simulink model "mars_rover_ex_1b"  (R2023a)
settings: Solver=ode23t  StartTime=0.0  StopTime=Rover.simStopTimeEx1b  FixedStep=1e-2  MaxStep=0.1  RelTol=1e-3  AbsTol=1e-3  EnableMultiTasking=on
StartFcn:
  | mars_rover_ex1b_sim_callback
model workspace (MATLAB code in the model file):
  | addpath("mars_rover_helpers");
  | % Load Rover Arm model for IK
  | mdlpath = ['mars_rover_data',filesep,'mars_rover_arm'];
  | load_system(mdlpath);
  | 
  | imdata = zeros(3,3,3);
  | 
  | % Temp
  | Kp_steer = 1;
  | Ki_steer = 1;
  | Kd_steer = 1;
  | 
  | Kp = 1;
  | Ki = 1;
  | Kd = 1;
values from neighbouring files (symbols this model uses):
  cam_base_angle = 0    [mars_rover_params.m]
  cam_target_angle = 20    [mars_rover_params.m]
  mapData = false(197,200)    [mars_rover_params.m]    (also in mars_rover_startup.m)
  roverPath = app.rover_path    [NavigateOnMars.m]    (also in mars_rover_params.m = rover_path1)
undefined symbols (not defined in the file or in its folder): Arm, armJointAng, armJointTrqs, cameraData, eeConfig, pose, Rover, rover_path_ex1, sampleLocation, steerAng, steerTrqs, Terrain, vSpeed, Wheel1_G, Wheel2_G, Wheel3_G, Wheel4_G, Wheel5_G, Wheel6_G, wheelTrqs, wSpeeds, X, Y, Z
libraries: sm_lib x238, nesl_utility x80, slpidlib x3, simulink x3, simulink_extras x2, robotcorelib x1, robotalgslib x1
(part 1 of 9)
settings Model: PacingRate=4  Creator=The MathWorks, Inc.
settings SolverCC: AutoScaleAbsTol=off  ZeroCrossAlgorithm=Adaptive  AlgebraicLoopSolver=TrustRegion  MinimalZcImpactIntegration=on  MaxZcPerStep=1
settings DataIOCC: MaxDataPoints=10000  SaveFormat=Array  ReturnWorkspaceOutputsName=sm_mars_rover_out_ex1b
settings OptimizationCC: LifeSpan=inf
settings DebuggingCC: IgnoredZcDiagnostic=none  UnconnectedInputMsg=warning  UnconnectedOutputMsg=warning  UnconnectedLineMsg=warning  AllowSymbolicDim=off  SFUnexpectedBacktrackingDiag=warning  SFNoUnconditionalDefaultTransitionDiag=warning  SFExecutionAtInitializationDiag=none  ArithmeticOperatorsInVariantConditions=warning
settings ModelReferenceCC: EnableRefExpFcnMdlSchedulingChecks=on
settings SFSimCC: SimUseLocalCustomCode=off  CustomCodeUndefinedFunction=UseInterfaceOnly
settings RTWCC: RTWUseLocalCustomCode=off  DLArmComputeVersion=19.05
settings CodeAppCC: StateflowObjectComments=on
settings GRTTargetCC: TargetLangStandard=C89/C90 (ANSI)
settings ConfigComp: CovMetricSettings=dw  CovSaveCumulativeToWorkspaceVar=on  CovSaveSingleToWorkspaceVar=on  CovExternalEMLEnable=off  CovSFcnEnable=off
settings SimscapeCC: SimscapeLogType=all  SimscapeLogSimulationStatistics=on  SimscapeLogName=simlog_sm_mars_rover  SimscapeLogLimitData=off  SimscapeLogDataHistory=10000
settings DiagnosticsConfigSet: SimMechanicsUnconnectedFramePorts=none  SimMechanicsUnconnectedGeometryPorts=none  SimMechanicsConflictingReferenceFrames=none
settings ExplorerConfigSet: SimMechanicsOpenEditorOnUpdate=off  InternalSimMechanicsExplorerSettings="<ExplorerConfiguration><canonicalview>default</canonicalview><AnimationSetting><BasePlaybackSpeed>1.0</BasePlaybackSpeed><PlaybackSpeedFactor>16.0</PlaybackSpeedFactor></AnimationSetting><TilePanel><TileInfo><Tiles Columns=\"1\" Count=\"1\" Rows=\"1\"><Column Weight=\"1\"/><Row Weight=\"1\"/><Tile Height=\"1\" Width=\"1\" X=\"0\" Y=\"0\"/></Tiles></TileInfo><SceneInfo><SceneViewer><BGColor><R>0.819607853889465332</R><G>0.709803938865661621</G><B>0.662745118141174316</B></BGColor><Camera><DoPerspective>on</DoPerspective><Position><X>20.0000024966346217</X><Y>19.6116525700285997</Y><Z>47.9479667849964954</Z></Position><Center><X>20.0000024966346217</X><Y>19.6116525700285997</Y><Z>2.96310309448505915</Z></Center><Up><X>0</X><Y>1</Y><Z>-0</Z></Up><ViewLimDist>1</ViewLimDist><YLim>0.466307658154998583</YLim><XLim>0.817592760631764226</XLim></Camera></SceneViewer></SceneInfo></TilePanel><MechEditorPanel><Cameras><Camera><Id>Camera1</Id><Value><Name>Rover_Free_View</Name><NativeCamera><PositionKeyframeSet/><CenterKeyframeSet/><UpVectorKeyframeSet/></NativeCamera></Value></Camera><Camera><Id>Camera6</Id><Value><Name>Rover_Right_ViewA</Name><NativeCamera><PositionTrackingFeature>Mars_Rover.Rover_Plant_Model_And_Control.Rover.Chassis.Chasis_Camera_RightA.R</PositionTrackingFeature><CenterTrackingFeature>Mars_Rover.Rover_Plant_Model_And_Control.Rover.Chassis.Chasis_Camera_RightA.R</CenterTrackingFeature><UpVectorTrackingFeature>Mars_Rover.Rover_Plant_Model_And_Control.Rover.Chassis.Chasis_Camera_RightA.R</UpVectorTrackingFeature><CenterTrackingOrigin>off</CenterTrackingOrigin><CenterTrackingDirection>+X</CenterTrackingDirection><UpVectorTrackingDirection>+Z</UpVectorTrackingDirection></NativeCamera></Value></Camera><Camera><Id>Camera7</Id><Value><Name>Rover_Rear_View</Name><NativeCamera><PositionTrackingFeature>Mars_Rover.Rover_Plant_Model_And_Control.Rover.Chassis.Chasis_Camera_Rear.R</PositionTrackingFeature><CenterTrackingFeature>Mars_Rover.Rover_Plant_Model_And_Control.Rover.Chassis.Chasis_Camera_Rear.R</CenterTrackingFeature><UpVectorTrackingFeature>Mars_Rover.Rover_Plant_Model_And_Control.Rover.Chassis.Chasis_Camera_Rear.R</UpVectorTrackingFeature><CenterTrackingOrigin>off</CenterTrackingOrigin><CenterTrackingDirection>-Y</CenterTrackingDirection><UpVectorTrackingDirection>+Z</UpVectorTrackingDirection></NativeCamera></Value></Camera><Camera><Id>Camera8</Id><Value><Name>Rover_Top_View</Name><NativeCamera><PositionTrackingFeature>Mars_Rover.Rover_Plant_Model_And_Control.Rover.Chassis.Chasis_Camera_Top.R</PositionTrackingFeature><CenterTrackingFeature>Mars_Rover.Rover_Plant_Model_And_Control.Rover.Chassis.Chasis_Camera_Top.R</CenterTrackingFeature><UpVectorTrackingFeature>Mars_Rover.Rover_Plant_Model_And_Control.Rover.Chassis.Chasis_Camera_Top.R</UpVectorTrackingFeature><CenterTrackingOrigin>off</CenterTrackingOrigin><CenterTrackingDirection>-Z</CenterTrackingDirection><UpVectorTrackingDirection>+X</UpVectorTrackingDirection></NativeCamera></Value></Camera><Camera><Id>Camera9</Id><Value><Name>Rover_Right_ViewB</Name><NativeCamera><PositionTrackingFeature>Mars_Rover.Rover_Plant_Model_And_Control.Rover.Chassis.Chasis_Camera_RightB.R</PositionTrackingFeature><CenterTrackingFeature>Mars_Rover.Rover_Plant_Model_And_Control.Rover.Chassis.Chasis_Camera_RightB.R</CenterTrackingFeature><UpVectorTrackingFeature>Mars_Rover.Rover_Plant_Model_And_Control.Rover.Chassis.Chasis_Camera_RightB.R</UpVectorTrackingFeature><CenterTrackingOrigin>off</CenterTrackingOrigin><CenterTrackingDirection>+X</CenterTrackingDirection><UpVectorTrackingDirection>+Z</UpVectorTrackingDirection></NativeCamera></Value></Camera><Camera><Id>Camera10</Id><Value><Name>RoverNavCamL</Name><NativeCamera><PositionTrackingFeature>Mars_Rover.Rover_Plant_Model_And_Control.Rover.Camera.rsm_head_1_RIGID.CameraFrameL.F</PositionTrackingFeature><CenterTrackingFeature>Mars_Rover.Rover_Plant_Model_And_Control.Rover.Camera.rsm_head_1_RIGID.CameraFrameL.F</CenterTrackingFeature><UpVectorTrackingFeature>Mars_Rover.Rover_Plant_Model_And_Control.Rover.Camera.rsm_head_1_RIGID.CameraFrameL.F</UpVectorTrackingFeature><CenterTrackingOrigin>off</CenterTrackingOrigin><CenterTrackingDirection>+X</CenterTrackingDirection><UpVectorTrackingDirection>+Z</UpVectorTrackingDirection></NativeCamera></Value></Camera><Camera><Id>Camera11</Id><Value><Name>RoverNavCamR</Name><NativeCamera><PositionTrackingFeature>Mars_Rover.Rover_Plant_Model_And_Control.Rover.Camera.rsm_head_1_RIGID.CameraFrameR.F</PositionTrackingFeature><CenterTrackingFeature>Mars_Rover.Rover_Plant_Model_And_Control.Rover.Camera.rsm_head_1_RIGID.CameraFrameR.F</CenterTrackingFeature><UpVectorTrackingFeature>Mars_Rover.Rover_Plant_Model_And_Control.Rover.Camera.rsm_head_1_RIGID.CameraFrameR.F</UpVectorTrackingFeature><CenterTrackingOrigin>off</CenterTrackingOrigin><CenterTrackingDirection>+X</CenterTrackingDirection><UpVectorTrackingDirection>+Z</UpVectorTrackingDirection></NativeCamera></Value></Camera></Cameras><GfxPanelCameraMap><MapElement CameraMLId=\"Camera10\" GfxPanelIndex=\"0\"/></GfxPanelCameraMap><VideoCreator><PlaybackSpeedRatio>8</PlaybackSpeedRatio><FrameRate>30</FrameRate><VideoFormat>MPEG-4</VideoFormat><FrameSize>[800 600]</FrameSize></VideoCreator></MechEditorPanel></ExplorerConfiguration>"

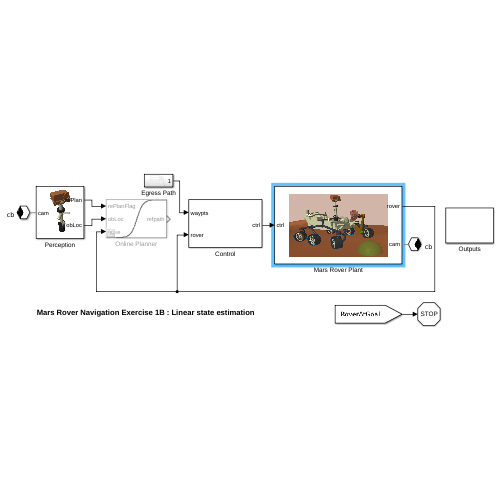
[thumbnail: Simulink's stored preview of the top-level diagram]
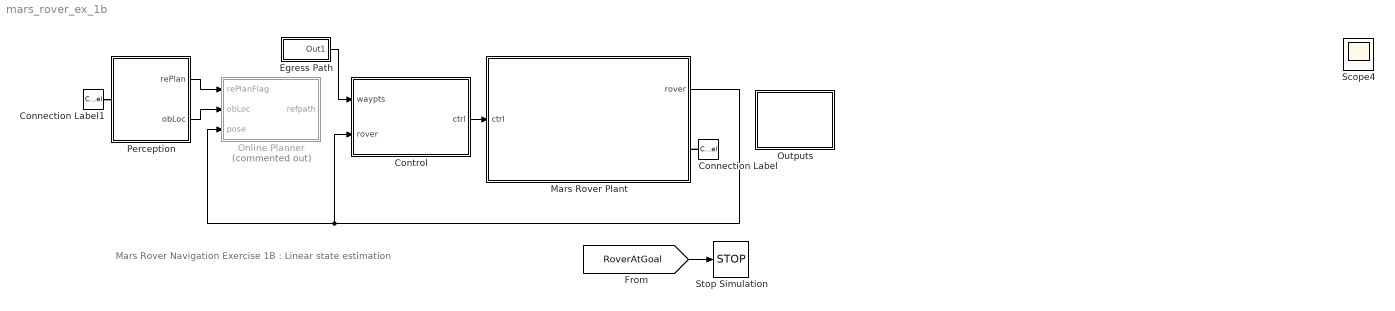
== system mars_rover_ex_1b ==
  note: Mars Rover Navigation Exercise 1B : Linear state estimation
  Connection Label : ConnectionLabel  Label=cb
  Connection Label1 : ConnectionLabel  Label=cb
  Control : Subsystem
  Egress Path : Subsystem
  Mars Rover Plant : Subsystem
      mask Display: image('$imagefile'); % Use "Edit Image" on toolstrip to change.
  Online Planner : Subsystem  Commented=on
      mask Display:
      | x = -5:0.01:5;
      | y = tanh(x);
      | plot(x,y)
  Outputs : Subsystem
  Perception : Subsystem
      mask Display: image('$imagefile'); % Use "Edit Image" on toolstrip to change.
  Stop Simulation : Stop
  Scope4 : Scope
  wires:
  Mars Rover Plant/1(rover) -> Online Planner/3(pose), Control/2(rover)
  Control/1(ctrl) -> Mars Rover Plant/1(ctrl)
  Perception/1(rePlan) -> Online Planner/1(rePlanFlag)
  Perception/2(obLoc) -> Online Planner/2(obLoc)
  Egress Path/1(Out1) -> Control/1(waypts)
  [RoverAtGoal] -> Stop Simulation/1
  connections:
  Connection Label/LConn1 -- Mars Rover Plant/RConn1
  Connection Label1/LConn1 -- Perception/LConn1

== system mars_rover_ex_1b/Control ==
  waypts : Inport
  rover : Inport  Port=2
  Bus Creator : BusCreator  Inputs=steerTrqs,wheelTrqs,armJointTrqs
  Bus Selector : BusSelector  OutputSignals=pose,vSpeed,steerAng,wSpeeds,sampleLocation,armJointAng
  Manipulator Control : Subsystem  Commented=on
  Rover Control : Subsystem
  ctrl : Outport
  wires:
  Bus Selector/3 -> Rover Control/4(ActSteerAng)  "<steerAng>"
  Bus Selector/6 -> Manipulator Control/2(ActJointAngles)  "<armJointAng>"
  Bus Selector/5 -> Manipulator Control/1(SampleLocation)  "<sampleLocation>"
  Bus Selector/2 -> Rover Control/3(vSpeed)  "<vSpeed>"
  Rover Control/2(WheelTrqs) -> Bus Creator/2  "wheelTrqs"
  Bus Selector/1 -> Rover Control/2(CurrentPose)  "<pose>"
  Bus Selector/4 -> Rover Control/5(ActWheelSpeed)  "<wSpeeds>"
  Rover Control/1(SteerTrqs) -> Bus Creator/1  "steerTrqs"
  Manipulator Control/1(y) -> Bus Creator/3  "armJointTrqs"
  rover/1 -> Bus Selector/1
  waypts/1 -> Rover Control/1(WayPts)
  Bus Creator/1 -> ctrl/1

== system mars_rover_ex_1b/Egress Path ==
  Constant : Constant  Value=rover_path_ex1.x
  Constant1 : Constant  Value=rover_path_ex1.y
  Matrix Concatenate : Concatenate  Mode=Multidimensional array  ConcatenateDimension=2
  Out1 : Outport
  wires:
  Constant/1 -> Matrix Concatenate/1
  Constant1/1 -> Matrix Concatenate/2
  Matrix Concatenate/1 -> Out1/1

== system mars_rover_ex_1b/Mars Rover Plant ==
  ctrl : Inport
  Bus Creator : BusCreator  Inputs=pose,vSpeed,steerAng,wSpeeds,armJointAng,sampleLocation
  Bus Selector : BusSelector  OutputSignals=steerTrqs,wheelTrqs,armJointTrqs
  DesRoverPathViz : Subsystem
  Manipulator Plant Model : Subsystem  Commented=on
      settings: PortSchema="{\"entries\":[{\"content\":{\"sides\":[{\"content\":{\"connectorIds\":[\"LConn1\",\"In1\"]},\"type\":\"ConnectorPlacement.EquallySpacedRectSide\",\"uuid\":\"1d5d5bba-8fe4-4512-81c9-941bf10e7a7e\"},{\"content\":{\"connectorIds\":[\"RConn1\",\"RConn2\",\"Out1\",\"Out2\"],\"side\":\"RIGHT\"},\"type\":\"ConnectorPlacement.EquallySpacedRectSide\",\"uuid\":\"9a182200-9de3-47d0-8b03-f46c5c0d90b9\"},{\"content\":{\"connectorIds\":[],\"side\":\"TOP\"},\"type\":\"ConnectorPlacement.EquallySpacedRectSide\",\"uuid\":\"d91c9a9a-8a5e-48c7-bbfb-96bbdec144af\"}]},\"type\":\"ConnectorPlacement.EquallySpacedConnector\",\"uuid\":\"893c2cf1-507c-408d-8167-3b555343645b\"}],\"packageUris\":[\"http://schema.mathworks.com/mf0/Connector/R2020b\"],\"version\":\"1.0\"}"
      mask Display:
      | image('RoverArmIcon.png'); % Use "Edit Image" on toolstrip to change.
      | 
      | color('black');
      | port_label('RConn',1,' sd','interpreter','tex')
      | port_label('LConn',1,' sb','interpreter','tex')
      | port_label('RConn',2,' armB','interpreter','tex')
      | port_label('output', 1, 'angles');
      | port_label('output', 2, 'sample');
      | port_label('input', 1, 'trqs');
  Rover Plant Model : Subsystem
      mask Display:
      | image('RoverIcon.PNG');
      | %image('$imagefile'); % Use "Edit Image" on toolstrip to change.
      | 
      | color('black');
      | port_label('LConn',1,' ref','interpreter','tex')
      | port_label('RConn',1,' armB','interpreter','tex')
      | port_label('RConn',2,' SD','interpreter','tex')
      | port_label('RConn',3,' CB','interpreter','tex')
      | port_label('output', 1, 'pose');
      | port_label('output', 2, 'vSpeed');
      | port_label('output', 3, 'sAng');
      | port_label('output', 4, 'wSpeed');
      | port_label('input', 1, 'sTrqs');
      | port_label('input', 2, 'wTrqs');
  cam : PMIOPort  Side=Right
  rover : Outport
  wires:
  Bus Selector/1 -> Rover Plant Model/1(Input)  "<steerTrqs>"
  Bus Selector/2 -> Rover Plant Model/2(Input1)  "<wheelTrqs>"
  Rover Plant Model/1(Pose) -> Bus Creator/1  "pose"
  Rover Plant Model/2(actRoverSpeed) -> Bus Creator/2  "vSpeed"
  Rover Plant Model/4(actWheelSpeeds) -> Bus Creator/4  "wSpeeds"
  Manipulator Plant Model/1(armJointAng) -> Bus Creator/5  "armJointAng"
  Manipulator Plant Model/2(sampleLocation) -> Bus Creator/6  "sampleLocation"
  Bus Selector/3 -> Manipulator Plant Model/1(Input)  "<armJointTrqs>"
  Bus Creator/1 -> rover/1
  Rover Plant Model/3(actSteerAng) -> Bus Creator/3  "steerAng"
  ctrl/1 -> Bus Selector/1
  connections:
  Rover Plant Model/LConn1 -- Manipulator Plant Model/LConn1 -- DesRoverPathViz/LConn1
  Rover Plant Model/RConn1 -- Manipulator Plant Model/RConn2
  Rover Plant Model/RConn2 -- Manipulator Plant Model/RConn1
  cam/RConn1 -- Rover Plant Model/RConn3

== system mars_rover_ex_1b/Online Planner ==
  rePlanFlag : Inport
  obLoc : Inport  Port=2
  pose : Inport  Port=3
  Bus Selector : BusSelector  OutputSignals=pose
  Constant13 : Constant  Value=[roverPath.x(end) roverPath.y(end) 0]
  Constant2 : Constant  Value=[roverPath.x roverPath.y]
  Online Planner : Subsystem
  Triggered Subsystem1 : Subsystem  TreatAsAtomicUnit=on
  Unit Delay : UnitDelay  InitialCondition=mapData  SampleTime=-1  HasFrameUpgradeWarning=on
  refpath : Outport
  tag scope: RefPath=global, mapData=global
  wires:
  Constant13/1 -> Online Planner/3(endLocation)
  Unit Delay/1 -> Online Planner/1(mapData)
  rePlanFlag/1 -> Triggered Subsystem1/Trigger, Online Planner/Trigger
  Triggered Subsystem1/1(Out1) -> Online Planner/2(startLocation)
  Online Planner/1(refpath) -> [RefPath], refpath/1
  pose/1 -> Bus Selector/1
  Bus Selector/1 -> Triggered Subsystem1/1(startLocation)  "<pose>"
  Constant2/1 -> Online Planner/5(initialRoverPath)
  Online Planner/2(newMapData) -> Unit Delay/1, [mapData]
  obLoc/1 -> Online Planner/4(obstacleLocation)

== system mars_rover_ex_1b/Outputs ==
  Rover Outputs : Subsystem

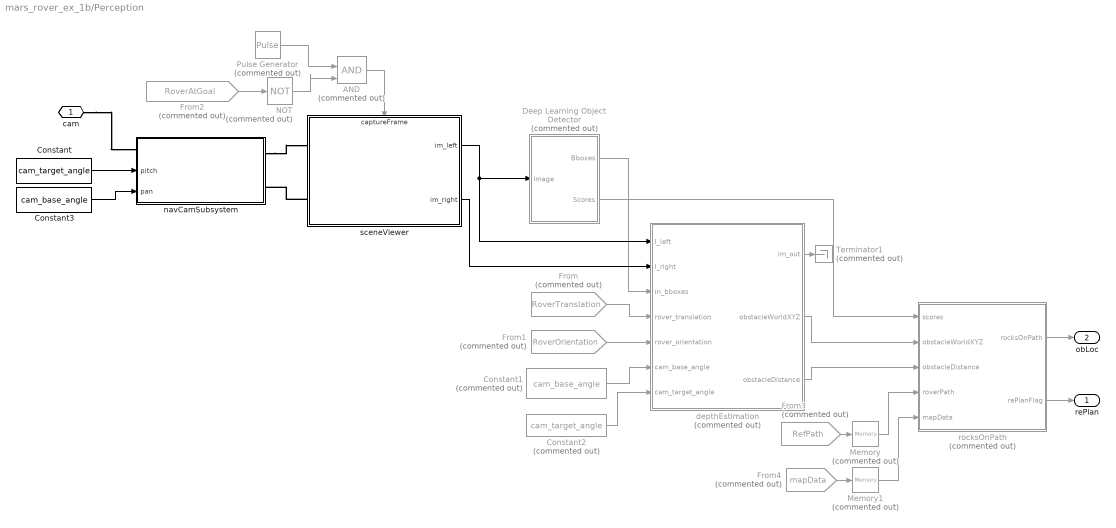
== system mars_rover_ex_1b/Perception ==
  AND : Logic  Commented=on  IconShape=distinctive  AllPortsSameDT=off  OutDataTypeStr=boolean
  Constant : Constant  Value=cam_target_angle
  Constant1 : Constant  Commented=on  Value=cam_base_angle
  Constant2 : Constant  Commented=on  Value=cam_target_angle
  Constant3 : Constant  Value=cam_base_angle
  Deep Learning Object Detector : Subsystem  Commented=on  mask(Deep Learning Object Detector){Detector=Detector from MAT-file, DetectorFunction=untitled, DetectorFilePath=rockDetectorDL.mat, MaxDetections=500, Bboxes=on, Labels=off, Scores=on, UseROI=off, ROI=[1 1 100 100], Threshold=0.8, NumStrongestRegions=2000, UseMinSize=off, MinSize=[1 1], UseMaxSize=off, MaxSize=[50 50], ForceInterpretedSim=off}
      mask prompts: Detector "vision:ObjectDetectorBlock:Detector"; DetectorFunction "vision:ObjectDetectorBlock:MatlabFunction"; DetectorFilePath "vision:ObjectDetectorBlock:FilePath"; MaxDetections "vision:ObjectDetectorBlock:MaxDetections"; Bboxes "vision:ObjectDetectorBlock:Bboxes"; Labels "vision:ObjectDetectorBlock:Labels"; Scores "vision:ObjectDetectorBlock:Scores"; UseROI "vision:ObjectDetectorBlock:UseROI"; Threshold "vision:ObjectDetectorBlock:Threshold"; NumStrongestRegions "vision:ObjectDetectorBlock:NumStrongestRegions"; UseMinSize "vision:ObjectDetectorBlock:UseMinSize"; UseMaxSize "vision:ObjectDetectorBlock:UseMaxSize"; ForceInterpretedSim "vision:ObjectDetectorBlock:ForceInterpretedSim"
      mask help: vision:ObjectDetectorBlock:Description
      mask init:
      | vision.internal.blocks.objectDetectorBlockWrapper(...
      |     'deep.blocks.internal.configureObjectDetector', ...
      |     gcb, ...
      |     bdroot, ...
      |     Detector, ...
      |     DetectorFilePath, ...
      |     DetectorFunction, ...
      |     logical(UseROI), ...
      |     ROI, ...
      |     Threshold, ...
      |     NumStrongestRegions, ...
      |     logical(UseMinSize), ...
      |     MinSize, ...
      |     logical(UseMaxSize), ...
      |     MaxSize, ...
      |     MaxDetections, ...
      |     logical(Bboxes), ...
      |     logical(Labels), ...
      |     logical(Scores), ...
      |     logical(ForceInterpretedSim));
      mask Help: helpview('vision', 'nnet_model_detect')
      mask TypeOptions Detector: vision:ObjectDetectorBlock:DetectorFromMatFile | vision:ObjectDetectorBlock:DetectorFromFunction
      mask Callback Detector: vision.internal.blocks.objectDetectorBlockWrapper('deep.blocks.internal.setNetworkSelectVisibility',gcb);
      mask Callback DetectorFunction: vision.internal.blocks.objectDetectorBlockWrapper('deep.blocks.internal.setObjectDetectorOptionsVisibility', gcb);
      mask Callback DetectorFilePath: vision.internal.blocks.objectDetectorBlockWrapper('deep.blocks.internal.setObjectDetectorOptionsVisibility', gcb);
      mask Callback UseROI: vision.internal.blocks.objectDetectorBlockWrapper('deep.blocks.internal.setEnabledParameterVisibility', gcb, 'UseROI', 'ROI');
      mask Callback UseMinSize: vision.internal.blocks.objectDetectorBlockWrapper('deep.blocks.internal.setEnabledParameterVisibility', gcb, 'UseMinSize', 'MinSize');
      mask Callback UseMaxSize: vision.internal.blocks.objectDetectorBlockWrapper('deep.blocks.internal.setEnabledParameterVisibility', gcb, 'UseMaxSize', 'MaxSize');
      mask DialogControl Detector Prompt: Detector:
      mask DialogControl DetectorFunction Prompt: MATLAB function:
      mask DialogControl DetectorFilePath Prompt: File path:
      mask DialogControl BrowseButton Prompt: vision:ObjectDetectorBlock:Browse
      mask DialogControl BrowseButton Callback: vision.internal.blocks.objectDetectorBlockWrapper('deep.blocks.internal.handleBrowseButtonClick', gcb);
      mask DialogControl OutputsTab Prompt: vision:ObjectDetectorBlock:Outputs
      mask DialogControl OutputsSizeGroup Prompt: vision:ObjectDetectorBlock:OutputsSize
      mask DialogControl MaxDetections Prompt: Maximum number of detections:
      mask DialogControl OutputPortsGroup Prompt: vision:ObjectDetectorBlock:OutputPorts
      mask DialogControl Bboxes Prompt: Bounding boxes
      mask DialogControl AdvancedTab Prompt: vision:ObjectDetectorBlock:Advanced
      mask DialogControl AdvancedParametersGroup Prompt: vision:ObjectDetectorBlock:AdvancedParameters
      mask DialogControl UseROI Prompt: Specify region of interest
      mask DialogControl Threshold Prompt: Detection threshold:
      mask DialogControl NumStrongestRegions Prompt: Number of strongest regions:
      mask DialogControl UseMinSize Prompt: Specify minimum region size
      mask DialogControl UseMaxSize Prompt: Specify maximum region size
      mask DialogControl HiddenContainer Prompt: Hidden Parameters
      mask DialogControl ForceInterpretedSim Prompt: Force interpreted simulation
  From : From  Commented=on  GotoTag=RoverTranslation  TagVisibility=global
  From1 : From  Commented=on  GotoTag=RoverOrientation  TagVisibility=global
  From2 : From  Commented=on  GotoTag=RoverAtGoal  TagVisibility=global
  From3 : From  Commented=on  GotoTag=RefPath  TagVisibility=global
  From4 : From  Commented=on  GotoTag=mapData  TagVisibility=global
  Memory : Memory  Commented=on  InitialCondition=[roverPath.x roverPath.y]
  Memory1 : Memory  Commented=on  InitialCondition=mapData
  NOT : Logic  Commented=on  Operator=NOT  IconShape=distinctive  AllPortsSameDT=off  OutDataTypeStr=boolean
  Pulse Generator : DiscretePulseGenerator  Commented=on  PulseType=Time based  Period=10000
  Terminator1 : Terminator  Commented=on
  depthEstimation : MATLAB Function  Commented=on  TreatAsAtomicUnit=on
  navCamSubsystem : Subsystem
      settings: PortSchema="{\"entries\":[{\"content\":{\"sides\":[{\"content\":{\"connectorIds\":[\"LConn1\",\"In1\",\"In2\"]},\"type\":\"ConnectorPlacement.EquallySpacedRectSide\",\"uuid\":\"2deb6c0b-0fb4-445b-86e3-b1fc7203c2ed\"},{\"content\":{\"connectorIds\":[\"RConn1\",\"RConn2\"],\"side\":\"RIGHT\"},\"type\":\"ConnectorPlacement.EquallySpacedRectSide\",\"uuid\":\"96d5d272-26bd-434a-b8d4-4dbdb87bfabc\"},{\"content\":{\"connectorIds\":[],\"side\":\"TOP\"},\"type\":\"ConnectorPlacement.EquallySpacedRectSide\",\"uuid\":\"0dc7d8f3-f281-4d7b-afc7-28fa8d470391\"}]},\"type\":\"ConnectorPlacement.EquallySpacedConnector\",\"uuid\":\"c3c449fe-5a97-4f9a-be85-0bfbae61164d\"}],\"packageUris\":[\"http://schema.mathworks.com/mf0/Connector/R2020b\"],\"version\":\"1.0\"}"
  rocksOnPath : MATLAB Function  Commented=on  TreatAsAtomicUnit=on
  sceneViewer : Subsystem
      settings: PortSchema="{\"entries\":[{\"content\":{\"sides\":[{\"content\":{\"connectorIds\":[\"LConn1\",\"LConn2\"]},\"type\":\"ConnectorPlacement.EquallySpacedRectSide\",\"uuid\":\"3e389f59-5740-42d0-b219-868887290247\"},{\"content\":{\"connectorIds\":[\"Out1\",\"Out2\"],\"side\":\"RIGHT\"},\"type\":\"ConnectorPlacement.EquallySpacedRectSide\",\"uuid\":\"8071baf0-f328-4328-afc3-7bbca75f94e9\"},{\"content\":{\"connectorIds\":[\"In1\"],\"side\":\"TOP\"},\"type\":\"ConnectorPlacement.EquallySpacedRectSide\",\"uuid\":\"389ad39b-6a15-4fbe-92ae-3d1bb225264a\"}]},\"type\":\"ConnectorPlacement.EquallySpacedConnector\",\"uuid\":\"9ad84bbc-3c32-4f8f-82ec-510eaa24821f\"}],\"packageUris\":[\"http://schema.mathworks.com/mf0/Connector/R2020b\"],\"version\":\"1.0\"}"
  cam : PMIOPort  Side=Left
  rePlan : Outport
  obLoc : Outport  Port=2
  wires:
  Deep Learning Object Detector/1(Bboxes) -> depthEstimation/3(in_bboxes)
  depthEstimation/2(obstacleWorldXYZ) -> rocksOnPath/2(obstacleWorldXYZ)
  depthEstimation/1(im_out) -> Terminator1/1
  From/1 -> depthEstimation/4(rover_translation)
  From1/1 -> depthEstimation/5(rover_orientation)
  Constant1/1 -> depthEstimation/6(cam_base_angle)
  Constant2/1 -> depthEstimation/7(cam_target_angle)
  From2/1 -> NOT/1
  NOT/1 -> AND/2
  rocksOnPath/1(rocksOnPath) -> obLoc/1
  rocksOnPath/2(rePlanFlag) -> rePlan/1
  Pulse Generator/1 -> AND/1
  From3/1 -> Memory/1
  Memory/1 -> rocksOnPath/4(roverPath)
  From4/1 -> Memory1/1
  Memory1/1 -> rocksOnPath/5(mapData)
  depthEstimation/3(obstacleDistance) -> rocksOnPath/3(obstacleDistance)
  Deep Learning Object Detector/2(Scores) -> rocksOnPath/1(scores)
  sceneViewer/1(im_left) -> Deep Learning Object Detector/1(Image), depthEstimation/1(I_left)
  AND/1 -> sceneViewer/1(captureFrame)
  sceneViewer/2(im_right) -> depthEstimation/2(I_right)
  Constant/1 -> navCamSubsystem/1(pitch)
  Constant3/1 -> navCamSubsystem/2(pan)
  connections:
  navCamSubsystem/RConn1 -- sceneViewer/LConn1
  sceneViewer/LConn2 -- navCamSubsystem/RConn2
  cam/RConn1 -- navCamSubsystem/LConn1

== system mars_rover_ex_1b/Control/Manipulator Control ==
  SampleLocation : Inport
  ActJointAngles : Inport  Port=2
  " Trajectory Planner" : Subsystem
  Add : Sum  Inputs=+-
  PID Control : slpidlib/PID Controller  Controller=PID  Form=Parallel  TimeDomain=Continuous-time  UseExternalTs=off  SampleTime=-1  IntegratorMethod=Forward Euler  FilterMethod=Forward Euler  ControllerParametersSource=internal  P=Arm.Kp_arm  I=Arm.Ki_arm  UseKiTs=off  D=Arm.Kd_arm  N=100  UseFilter=on  TunerSelectOption=Transfer Function Based (PID Tuner App)  InitialConditionSource=internal  InitialConditionForIntegrator=0  InitialConditionForFilter=0  DifferentiatorICPrevScaledInput=0  ExternalReset=none  TrackingMode=off  Kt=1  LimitOutput=off  SatLimitsSource=internal  UpperSaturationLimit=inf  LowerSaturationLimit=-inf  LinearizeAsGain=on  AntiWindupMode=none  Kb=1  POutMin=[]  POutMax=[]  IOutMin=[]  IOutMax=[]  DOutMin=[]  DOutMax=[]  NOutMin=[]  NOutMax=[]  SumOutMin=[]  SumOutMax=[]  SaturationOutMin=[]  SaturationOutMax=[]  PParamMin=[]  PParamMax=[]  IParamMin=[]  IParamMax=[]  DParamMin=[]  DParamMax=[]  NParamMin=[]  NParamMax=[]  KbParamMin=[]  KbParamMax=[]  KtParamMin=[]  KtParamMax=[]  KbOutMin=[]  KbOutMax=[]  KtOutMin=[]  KtOutMax=[]  IntegratorOutMin=[]  IntegratorOutMax=[]  FilterOutMin=[]  FilterOutMax=[]  SumI1OutMin=[]  SumI1OutMax=[]  SumI2OutMin=[]  SumI2OutMax=[]  SumI3OutMin=[]  SumI3OutMax=[]  SumI4OutMin=[]  SumI4OutMax=[]  SumDOutMin=[]  SumDOutMax=[]  DifferentiatorOutMin=[]  DifferentiatorOutMax=[]  FilterDiffOutCoefMin=[]  FilterDiffOutCoefMax=[]  ReciprocalOutMin=[]  ReciprocalOutMax=[]  SumDenOutMin=[]  SumDenOutMax=[]  SumNumOutMin=[]  SumNumOutMax=[]  DivideOutMin=[]  DivideOutMax=[]  UdiffTsProdOutMin=[]  UdiffTsProdOutMax=[]  NTsProdOutMin=[]  NTsProdOutMax=[]  UintegralTsProdOutMin=[]  UintegralTsProdOutMax=[]  UngainTsProdOutMin=[]  UngainTsProdOutMax=[]  IntegratorContinuousStateAttributes=''  IntegratorStateMustResolveToSignalObject=off  IntegratorRTWStateStorageClass=Auto  FilterContinuousStateAttributes=''  FilterStateMustResolveToSignalObject=off  FilterRTWStateStorageClass=Auto  ParallelPVariant=InternalParameters  IdealPVariant=Disabled  IVariant=InternalParameters  DVariant=InternalParameters  IntegratorVariant=Continuous  SatVariant=Disabled  AWVariant=Passthrough  PCopyVariant=Disabled  TRVariant=Disabled  FdbkBlocksVariant=Forward  IdealPFdbkVariant=Disabled  SatFdbkVariant=Disabled  DerivativeFilterVariant=ContFilter  NVariant=InternalParameters  NCopyVariant=Disabled  FilterICVariant=InternalICsFilter  IntegratorICVariant=InternalICs  ExternalResetVariant=Disabled  TRSumVariant=Passthrough  SumFdbkVariant=Disabled  SumVariant=Sum_PID  TsampFilterVariant=InternalTs  TsampNgainVariant=Passthrough  TsampIntegralVariant=Passthrough  ExternalSaturationOutDataTypeStr=Inherit: Same as second input
  y : Outport
  tag scope: ActJointAngles=global, DesiredJointAngles=global, JointActuatorTrqs=global
  wires:
  PID Control/1 -> y/1, [JointActuatorTrqs]
  SampleLocation/1 -> " Trajectory Planner"/1(SampleLocation)
  ActJointAngles/1 -> Add/2, [ActJointAngles], " Trajectory Planner"/2(ActJointAngles)
  " Trajectory Planner"/1(DesiredJointAngles) -> Add/1, [DesiredJointAngles]
  Add/1 -> PID Control/1

== system mars_rover_ex_1b/Control/Rover Control ==
  WayPts : Inport
  CurrentPose : Inport  Port=2
  vSpeed : Inport  Port=3
  ActSteerAng : Inport  Port=4
  ActWheelSpeed : Inport  Port=5
  Rover Path Planning And Control : Subsystem
  Steering Controller : Subsystem
  Wheel Speed Controller : Subsystem
  SteerTrqs : Outport
  WheelTrqs : Outport  Port=2
  wires:
  Rover Path Planning And Control/2(DesWheelSpeeds) -> Wheel Speed Controller/1(DesWheelSpeeds)
  ActWheelSpeed/1 -> Wheel Speed Controller/2(ActWheelSpeed)
  Rover Path Planning And Control/1(DesSteerAngs) -> Steering Controller/1(DesSteerAng)
  CurrentPose/1 -> Rover Path Planning And Control/2(CurrentPose)
  Steering Controller/1(SteerTrqs) -> SteerTrqs/1
  ActSteerAng/1 -> Steering Controller/2(ActSteerAng)
  vSpeed/1 -> Rover Path Planning And Control/3(vSpeed)
  Wheel Speed Controller/1(WheelTrqs) -> WheelTrqs/1
  WayPts/1 -> Rover Path Planning And Control/1(WayPts)

== system mars_rover_ex_1b/Mars Rover Plant/DesRoverPathViz ==
  Cylindrical Solid : sm_lib/Body Elements/Cylindrical Solid  Commented=on  GraphicAmbientColor=[0.15 0.15 0.15 1.0]  BasedOnType=Density  CenterOfMass=[0 0 0]  CenterOfMassUnits=m  GraphicDiffuseColor=[0.4 0.4 1.0]  CylinderLength=0.1  CylinderLengthUnits=m  CylinderRadius=1  CylinderRadiusUnits=m  Density=1000  DensityUnits=kg/m^3  DoExposeReferenceFrame=on  GraphicEmissiveColor=[0.0 0.0 0.0 1.0]  ExportEntireGeometry=off  SerializedFrames=<Frames/>  MarkerShape=Sphere  MarkerSize=10  GraphicType=FromGeometry  InertiaType=CalculateFromGeometry  Mass=1  MassUnits=kg  MomentsOfInertia=[1 1 1]  MomentsOfInertiaUnits=kg*m^2  GraphicOpacity=0.5  ProductsOfInertia=[0 0 0]  ProductsOfInertiaUnits=kg*m^2  GraphicShininess=75  GraphicSpecularColor=[0.5 0.5 0.5 1.0]  GraphicVisPropType=SimpleVisualProperties
  Desired Path Viz : sm_lib/Curves and Surfaces/Point Cloud  Commented=on  CoordinatesMatrix=point_cloud_path_ex1  CoordinatesMatrixUnits=m  GraphicType=MarkerCloud  GraphicSphereRadius=0.05  GraphicSphereRadiusUnits=m  GraphicVisPropType=SimpleVisualProperties  GraphicDiffuseColor=[0 0 1]  GraphicOpacity=0.5  GraphicSpecularColor=[0.5 0.5 0.5 1.0]  GraphicAmbientColor=[0.15 0.15 0.15 1.0]  GraphicEmissiveColor=[0.0 0.0 0.0 1.0]  GraphicShininess=75
  Mechanism Configuration : sm_lib/Utilities/Mechanism Configuration  UniformGravity=Constant  GravityVector=[0 0 -3.7]  GravityVectorUnits=m/s^2  LinearizationDelta=0.001  JointModeTransitionNonlinearIterations=2
  Rigid Transform1 : sm_lib/Frames and Transforms/Rigid Transform  Commented=on  TranslationMethod=Cartesian  TranslationStandardOffset=1.85  TranslationStandardOffsetUnits=m  TranslationStandardAxis=+Z  TranslationCartesianOffset=[roverPath.x(end) roverPath.y(end) roverPath.z(end)]  TranslationCartesianOffsetUnits=m  TranslationROffset=0  TranslationROffsetUnits=m  TranslationZOffset=0  TranslationZOffsetUnits=m  TranslationThetaOffset=0  TranslationThetaOffsetUnits=deg  RotationMethod=None  RotationAngleUnits=deg  RotationStandardAxis=+X  RotationAngle=90  RotationArbitraryAxis=[0 0 1]  FollAlignAxisA=+X  BaseAlignAxisA=+Y  FollAlignAxisB=+Y  BaseAlignAxisB=+Z  RotationSequenceAxes=FollowerAxes  RotationSequence=XYX  RotationSequenceAngles=[0 0 0]  RotationSequenceAnglesUnits=deg  RotationMatrix=[1 0 0; 0 1 0; 0 0 1]  Quaternion=[1 0 0 0]
  Rigid Transform6 : sm_lib/Frames and Transforms/Rigid Transform  Commented=on  TranslationMethod=Cartesian  TranslationStandardOffset=1.85  TranslationStandardOffsetUnits=m  TranslationStandardAxis=+Z  TranslationCartesianOffset=[0 0 0.05]  TranslationCartesianOffsetUnits=m  TranslationROffset=0  TranslationROffsetUnits=m  TranslationZOffset=0  TranslationZOffsetUnits=m  TranslationThetaOffset=0  TranslationThetaOffsetUnits=deg  RotationMethod=None  RotationAngleUnits=deg  RotationStandardAxis=+X  RotationAngle=90  RotationArbitraryAxis=[0 0 1]  FollAlignAxisA=+X  BaseAlignAxisA=+Y  FollAlignAxisB=+Y  BaseAlignAxisB=+Z  RotationSequenceAxes=FollowerAxes  RotationSequence=XYX  RotationSequenceAngles=[0 0 0]  RotationSequenceAnglesUnits=deg  RotationMatrix=[1 0 0; 0 1 0; 0 0 1]  Quaternion=[1 0 0 0]
  Solver Configuration : nesl_utility/Solver Configuration  PhysicalDomain=network_engine_domain  SubClassName=solver  LeftPortType=input  RightPortType=generic  Tones=[]  Harmonics=[]  SimulateNoise=off  Profile=off  UseLocalSampling=off  EnableSwitchedLinearOptims=on  FrequencyDomain=off  UseCCode=off  RelTol=0.001  AbsTol=1e-06  MinStep=1e-09  ToWorkspace=off  RevertToSquareIcSolve=off  NumHomotopyIterations=100  PhasorMode=off  PhasorModeNumHarmonics=1  ConsistencySolver=NEWTON_FTOL  IndexReductionMethod=DerivativeReplacement  DoDC=off  ResidualTolerance=1e-09  ConsistencyTolSource=GLOBAL  ConsistencyAbsTol=0.001  ConsistencyRelTol=0.001  ConsistencyTolFactor=0.001  UseLocalSolver=off  LocalSolverChoice=NE_BACKWARD_EULER_ADVANCER  ResolveIndetEquations=on  FunctionEvalNumThread=1  LocalSolverSampleTime=0.001  DoFixedCost=off  MaxNonlinIter=3  MaxModeIter=2  ComputeImpulses=off  ImpulseIterations=2  LinearAlgebra=auto  LinearAlgebraNumThread=0  EquationFormulation=NE_TIME_EF  DelaysMemoryBudget=1024  AutomaticFiltering=on  FilteringTimeConstant=0.001  PartitionStorageMethod=AS_NEEDED  PartitionMemoryBudget=1024  PartitionMethod=FAST
  World Frame : sm_lib/Frames and Transforms/World Frame
  R : PMIOPort  Side=Left
  connections:
  Rigid Transform1/LConn1 -- Rigid Transform6/RConn1 -- Desired Path Viz/LConn1
  Cylindrical Solid/RConn1 -- Rigid Transform1/RConn1
  R/RConn1 -- World Frame/RConn1 -- Solver Configuration/RConn1 -- Mechanism Configuration/RConn1 -- Rigid Transform6/LConn1

== system mars_rover_ex_1b/Mars Rover Plant/Manipulator Plant Model ==
  Input : Inport
  End Effector Sense : Subsystem
  Rover Arm : Subsystem
      mask Display: image('$imagefile'); % Use "Edit Image" on toolstrip to change.
  Sample Interaction Logic : Subsystem
      mask Display: image('$imagefile'); % Use "Edit Image" on toolstrip to change.
  Sample Loc Sense : Subsystem
  SampleGeneration : Subsystem
  RoverRef : PMIOPort  Side=Left
  SampleDrop : PMIOPort  Port=2  Side=Right
  ArmBase : PMIOPort  Port=3  Side=Right
  armJointAng : Outport
  sampleLocation : Outport  Port=2
  wires:
  Input/1 -> Rover Arm/1(ActuatorTrqs)
  Rover Arm/1(JointAngles) -> armJointAng/1
  Sample Loc Sense/1(SamplePos) -> sampleLocation/1
  connections:
  Sample Interaction Logic/RConn1 -- SampleDrop/RConn1
  End Effector Sense/RConn1 -- Sample Interaction Logic/LConn2 -- Rover Arm/RConn1
  Sample Interaction Logic/LConn3 -- Sample Loc Sense/RConn1
  ArmBase/RConn1 -- Sample Loc Sense/LConn1 -- End Effector Sense/LConn1 -- Rover Arm/LConn1
  SampleGeneration/LConn1 -- RoverRef/RConn1
  Sample Interaction Logic/LConn1 -- SampleGeneration/RConn1

== system mars_rover_ex_1b/Mars Rover Plant/Rover Plant Model ==
  Input : Inport
  Input1 : Inport  Port=2
  Rigid Terrain Surface : Subsystem
      mask Display: image('$imagefile'); % Use "Edit Image" on toolstrip to change.
  "Rover " : Subsystem
      settings: PortSchema="{\"entries\":[{\"content\":{\"sides\":[{\"content\":{\"connectorIds\":[\"In1\",\"In2\"]},\"type\":\"ConnectorPlacement.EquallySpacedRectSide\",\"uuid\":\"1e8a3e2b-b3ca-4467-863a-9c237d71771f\"},{\"content\":{\"connectorIds\":[\"RConn1\",\"Out1\",\"Out2\",\"RConn2\"],\"side\":\"RIGHT\"},\"type\":\"ConnectorPlacement.EquallySpacedRectSide\",\"uuid\":\"1c304fdb-ff64-4dc8-bd28-208b239a200a\"},{\"content\":{\"connectorIds\":[\"LConn1\",\"LConn2\",\"LConn3\"],\"side\":\"TOP\"},\"type\":\"ConnectorPlacement.EquallySpacedRectSide\",\"uuid\":\"6fd19973-5814-4525-bce6-20dd9c942e44\"},{\"content\":{\"connectorIds\":[],\"side\":\"BOTTOM\"},\"type\":\"ConnectorPlacement.EquallySpacedRectSide\",\"uuid\":\"ce53b395-dae7-4df5-bc94-fd3f2fb0670c\"}]},\"type\":\"ConnectorPlacement.EquallySpacedConnector\",\"uuid\":\"720db96a-3f3b-4ddd-a986-ea75ab459e47\"}],\"packageUris\":[\"http://schema.mathworks.com/mf0/Connector/R2020b\"],\"version\":\"1.0\"}"
      mask Display: image('$imagefile'); % Use "Edit Image" on toolstrip to change.
  Rover Pose Sensing : Subsystem
  Terminator : Terminator
  World Frame1 : sm_lib/Frames and Transforms/World Frame
  ArmB : PMIOPort  Side=Right
  SampleDropLoc : PMIOPort  Port=2  Side=Right
  B : PMIOPort  Port=3  Side=Left
  CB : PMIOPort  Port=4  Side=Right
  Pose : Outport
  actRoverSpeed : Outport  Port=2
  actSteerAng : Outport  Port=3
  actWheelSpeeds : Outport  Port=4
  wires:
  Rover Pose Sensing/3(vSpeed) -> actRoverSpeed/1
  "Rover "/1(ActSteerAng) -> actSteerAng/1
  "Rover "/2(ActWheelSpeeds) -> actWheelSpeeds/1
  Input/1 -> "Rover "/1(SteeringTrqs)
  Input1/1 -> "Rover "/2(WheelTrqs)
  Rover Pose Sensing/1(estimatedPose) -> Pose/1
  Rover Pose Sensing/2(Pose) -> Terminator/1
  connections:
  ArmB/RConn1 -- "Rover "/LConn1
  SampleDropLoc/RConn1 -- "Rover "/LConn2
  World Frame1/RConn1 -- Rigid Terrain Surface/RConn1
  Rigid Terrain Surface/LConn1 -- "Rover "/RConn2
  Rover Pose Sensing/LConn2 -- "Rover "/RConn1
  B/RConn1 -- Rover Pose Sensing/LConn1
  CB/RConn1 -- "Rover "/LConn3

== system mars_rover_ex_1b/Online Planner/Online Planner ==
  mapData : Inport  OutDataTypeStr=boolean
  startLocation : Inport  Port=2
  endLocation : Inport  Port=3
  obstacleLocation : Inport  Port=4
  initialRoverPath : Inport  Port=5
  Trigger : TriggerPort  VariantControl=(inherit)
  pathPlanner : MATLAB Function  TreatAsAtomicUnit=on
  refpath : Outport  InitialOutput=[roverPath.x roverPath.y]
  newMapData : Outport  Port=2  InitialOutput=mapData
  correctedObsLoc : Outport  Port=3  InitialOutput=zeros(100,3)
  wires:
  obstacleLocation/1 -> pathPlanner/4(obstacleLocation)
  mapData/1 -> pathPlanner/1(mapData)
  startLocation/1 -> pathPlanner/2(startLocation)
  pathPlanner/1(refpath) -> refpath/1
  endLocation/1 -> pathPlanner/3(endLocation)
  initialRoverPath/1 -> pathPlanner/5(initRoverPath)
  pathPlanner/2(newMapData) -> newMapData/1
  pathPlanner/3(correctedObsLoc) -> correctedObsLoc/1

== system mars_rover_ex_1b/Online Planner/Triggered Subsystem1 ==
  startLocation : Inport
  Trigger : TriggerPort  VariantControl=(inherit)
  Out1 : Outport
  wires:
  startLocation/1 -> Out1/1

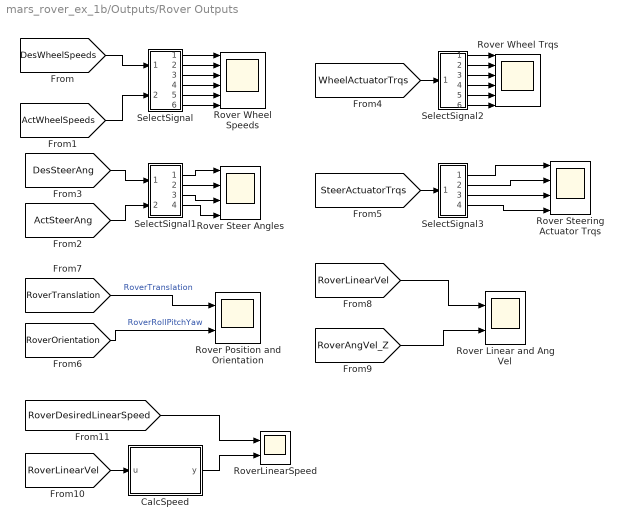
== system mars_rover_ex_1b/Outputs/Rover Outputs ==
  CalcSpeed : MATLAB Function  TreatAsAtomicUnit=on
  Rover Linear and Ang Vel : Scope  NumInputPorts=2
  Rover Position and Orientation : Scope  NumInputPorts=2
  Rover Steer Angles : Scope  NumInputPorts=4
  Rover Steering Actuator Trqs : Scope  NumInputPorts=4
  Rover Wheel Speeds : Scope  NumInputPorts=6
  Rover Wheel Trqs : Scope  NumInputPorts=6
  RoverLinearSpeed : Scope  NumInputPorts=2
  SelectSignal : Subsystem
  SelectSignal1 : Subsystem
  SelectSignal2 : Subsystem
  SelectSignal3 : Subsystem
  wires:
  CalcSpeed/1(y) -> RoverLinearSpeed/2
  SelectSignal3/1(Out1) -> Rover Steering Actuator Trqs/1
  [RoverLinearVel] -> CalcSpeed/1(u)
  [RoverAngVel_Z] -> Rover Linear and Ang Vel/2
  [RoverLinearVel] -> Rover Linear and Ang Vel/1
  [DesWheelSpeeds] -> SelectSignal/1(In1)
  SelectSignal2/4(Out4) -> Rover Wheel Trqs/4
  [WheelActuatorTrqs] -> SelectSignal2/1(In1)
  SelectSignal1/2(Out2) -> Rover Steer Angles/2
  [RoverTranslation] -> Rover Position and Orientation/1  "RoverTranslation"
  SelectSignal3/2(Out2) -> Rover Steering Actuator Trqs/2
  SelectSignal3/3(Out3) -> Rover Steering Actuator Trqs/3
  [DesSteerAng] -> SelectSignal1/1(In1)
  SelectSignal2/3(Out3) -> Rover Wheel Trqs/3
  [RoverOrientation] -> Rover Position and Orientation/2  "RoverRollPitchYaw"
  SelectSignal3/4(Out5) -> Rover Steering Actuator Trqs/4
  SelectSignal2/6(Out6) -> Rover Wheel Trqs/6
  SelectSignal/3(Out3) -> Rover Wheel Speeds/3
  SelectSignal2/5(Out5) -> Rover Wheel Trqs/5
  SelectSignal/1(Out1) -> Rover Wheel Speeds/1
  SelectSignal/6(Out6) -> Rover Wheel Speeds/6
  [ActWheelSpeeds] -> SelectSignal/2(In2)
  SelectSignal2/1(Out1) -> Rover Wheel Trqs/1
  SelectSignal1/4(Out5) -> Rover Steer Angles/4
  [ActSteerAng] -> SelectSignal1/2(In2)
  SelectSignal/2(Out2) -> Rover Wheel Speeds/2
  [SteerActuatorTrqs] -> SelectSignal3/1(In1)
  SelectSignal/5(Out4) -> Rover Wheel Speeds/5
  SelectSignal2/2(Out2) -> Rover Wheel Trqs/2
  SelectSignal/4(Out5) -> Rover Wheel Speeds/4
  SelectSignal1/1(Out1) -> Rover Steer Angles/1
  SelectSignal1/3(Out3) -> Rover Steer Angles/3
  [RoverDesiredLinearSpeed] -> RoverLinearSpeed/1

== system mars_rover_ex_1b/Perception/Deep Learning Object Detector ==
  Image : Inport
  MLFB : MATLAB Function  TreatAsAtomicUnit=on
  Bboxes : Outport
  Scores : Outport  Port=2
  wires:
  Image/1 -> MLFB/1(image)
  MLFB/1(bboxes) -> Bboxes/1
  MLFB/2(scores) -> Scores/1

== system mars_rover_ex_1b/Perception/navCamSubsystem ==
  pitch : Inport
  pan : Inport  Port=2
  Revolute Joint5 : sm_lib/Joints/Revolute Joint  JointMode=Normal  SenseConstraintForce=off  SenseConstraintForceX=off  SenseConstraintForceY=off  SenseConstraintForceZ=off  SenseConstraintTorque=off  SenseConstraintTorqueX=off  SenseConstraintTorqueY=off  SenseConstraintTorqueZ=off  SenseTotalForce=off  SenseTotalForceX=off  SenseTotalForceY=off  SenseTotalForceZ=off  SenseTotalTorque=off  SenseTotalTorqueX=off  SenseTotalTorqueY=off  SenseTotalTorqueZ=off  CompositeWrenchDir=FollowerOnBase  CompositeWrenchFrame=BaseFrame  EquilibriumPosition=0  EquilibriumPositionUnits=deg  SpringStiffness=0  SpringStiffnessUnits=N*m/deg  DampingCoefficient=0  DampingCoefficientUnits=N*m/(deg/s)  TorqueActuationMode=ComputedTorque  MotionActuationMode=InputMotion  SensePosition=off  SenseVelocity=off  SenseAcceleration=off  SenseTorqueForce=off  SenseLowerLimitTorqueForce=off  SenseUpperLimitTorqueForce=off  LowerLimitSpecify=off  LowerLimitBound=-90  LowerLimitBoundUnits=deg  LowerLimitStiffness=1e4  LowerLimitStiffnessUnits=N*m/deg  LowerLimitDamping=10  LowerLimitDampingUnits=N*m/(deg/s)  LowerLimitTransitionRegionWidth=0.1  LowerLimitTransitionRegionWidthUnits=deg  UpperLimitSpecify=off  UpperLimitBound=90  UpperLimitBoundUnits=deg  UpperLimitStiffness=1e4  UpperLimitStiffnessUnits=N*m/deg  UpperLimitDamping=10  UpperLimitDampingUnits=N*m/(deg/s)  UpperLimitTransitionRegionWidth=0.1  UpperLimitTransitionRegionWidthUnits=deg  PositionTargetSpecify=off  PositionTargetPriority=High  PositionTargetValue=0  PositionTargetValueUnits=deg  VelocityTargetSpecify=off  VelocityTargetPriority=High  VelocityTargetValue=0  VelocityTargetValueUnits=deg/s
  Rigid Transform1 : sm_lib/Frames and Transforms/Rigid Transform  TranslationMethod=None  TranslationStandardOffset=0  TranslationStandardOffsetUnits=m  TranslationStandardAxis=+Z  TranslationCartesianOffset=[0 0 0]  TranslationCartesianOffsetUnits=m  TranslationROffset=0  TranslationROffsetUnits=m  TranslationZOffset=0  TranslationZOffsetUnits=m  TranslationThetaOffset=0  TranslationThetaOffsetUnits=deg  RotationMethod=StandardAxis  RotationAngleUnits=deg  RotationStandardAxis=+X  RotationAngle=90  RotationArbitraryAxis=[0 0 1]  FollAlignAxisA=+X  BaseAlignAxisA=+Y  FollAlignAxisB=+Y  BaseAlignAxisB=+Z  RotationSequenceAxes=FollowerAxes  RotationSequence=XYX  RotationSequenceAngles=[0 0 0]  RotationSequenceAnglesUnits=deg  RotationMatrix=[1 0 0; 0 1 0; 0 0 1]  Quaternion=[1 0 0 0]
  Rigid Transform2 : sm_lib/Frames and Transforms/Rigid Transform  TranslationMethod=None  TranslationStandardOffset=0  TranslationStandardOffsetUnits=m  TranslationStandardAxis=+Z  TranslationCartesianOffset=[0 0 0]  TranslationCartesianOffsetUnits=m  TranslationROffset=0  TranslationROffsetUnits=m  TranslationZOffset=0  TranslationZOffsetUnits=m  TranslationThetaOffset=0  TranslationThetaOffsetUnits=deg  RotationMethod=StandardAxis  RotationAngleUnits=deg  RotationStandardAxis=+X  RotationAngle=-90  RotationArbitraryAxis=[0 0 1]  FollAlignAxisA=+X  BaseAlignAxisA=+Y  FollAlignAxisB=+Y  BaseAlignAxisB=+Z  RotationSequenceAxes=FollowerAxes  RotationSequence=XYX  RotationSequenceAngles=[0 0 0]  RotationSequenceAnglesUnits=deg  RotationMatrix=[1 0 0; 0 1 0; 0 0 1]  Quaternion=[1 0 0 0]
  Simulink-PS Converter : nesl_utility/Simulink-PS Converter  PhysicalDomain=network_engine_domain  SubClassName=ps_input  LeftPortType=input  RightPortType=output  PseudoPeriodic=off  Frequencies=[]  NoiseDistribution=none  NoiseParameters=[]  Unit=deg  AffineConversion=off  FilteringAndDerivatives=filter  SimscapeFilterOrder=2  InputFilterTimeConstant=0.001  UdotUserProvided=0
  rsm_base_1_RIGID : Subsystem
  rsm_head_1_RIGID : Subsystem
  rsm_lower_mast_2_RIGID : Subsystem
  rsm_outer_ring_1_RIGID : Subsystem
  rsm_upper_mast_1_RIGID : Subsystem
  CB : PMIOPort  Side=Left
  RightNavCam : PMIOPort  Port=2  Side=Right
  LeftNavCam : PMIOPort  Port=3  Side=Right
  wires:
  pitch/1 -> Simulink-PS Converter/1
  pan/1 -> rsm_upper_mast_1_RIGID/1(In1)
  connections:
  CB/RConn1 -- Rigid Transform1/LConn1
  Revolute Joint5/RConn1 -- Rigid Transform2/LConn1
  rsm_lower_mast_2_RIGID/RConn1 -- rsm_outer_ring_1_RIGID/LConn2
  Rigid Transform2/RConn1 -- rsm_base_1_RIGID/LConn1
  LeftNavCam/RConn1 -- rsm_head_1_RIGID/RConn2
  rsm_outer_ring_1_RIGID/LConn1 -- rsm_upper_mast_1_RIGID/LConn1
  rsm_lower_mast_2_RIGID/LConn1 -- rsm_base_1_RIGID/LConn2
  Revolute Joint5/LConn2 -- Simulink-PS Converter/RConn1
  Rigid Transform1/RConn1 -- Revolute Joint5/LConn1
  rsm_head_1_RIGID/LConn1 -- rsm_upper_mast_1_RIGID/RConn1
  rsm_head_1_RIGID/RConn1 -- RightNavCam/RConn1

== system mars_rover_ex_1b/Perception/sceneViewer ==
  captureFrame : Inport
  Left : Subsystem
  Right : Subsystem
  Stereo_Left : Subsystem  Commented=on
  Stereo_Right : Subsystem  Commented=on
  rightCamFrame : PMIOPort  Side=Left
  leftCamFrame : PMIOPort  Port=2  Side=Left
  im_left : Outport
  im_right : Outport  Port=2
  wires:
  Stereo_Right/1(im_right) -> im_right/1
  captureFrame/1 -> Stereo_Right/1(Input), Stereo_Left/1(Input)
  Stereo_Left/1(im_left) -> im_left/1
  connections:
  Stereo_Right/LConn1 -- rightCamFrame/RConn1 -- Right/RConn1
  Stereo_Left/LConn1 -- Left/RConn1 -- leftCamFrame/RConn1

== system mars_rover_ex_1b/Control/Manipulator Control/ Trajectory Planner ==
  SampleLocation : Inport
  ActJointAngles : Inport  Port=2
  Constant : Constant  Value="[-2.2294 -125.2918   50.0575 -175.3493  177.7706  180.0000]"
  Delay : Delay
  Delay1 : Delay  DelayLength=35
  Planner Subsystem : Subsystem
  SampleDropOffCmdLogic : Subsystem
  SampleLoc wrt arm base : Subsystem
  SamplePickUpCmdLogic : Subsystem
  Stop Simulation : Stop
  Switch : Switch  Criteria=u2 > Threshold  SaturateOnIntegerOverflow=off  InputSameDT=off
  DesiredJointAngles : Outport
  tag scope: SampleDropOffFlag=global, SamplePickFlag=global
  wires:
  Switch/1 -> DesiredJointAngles/1
  Constant/1 -> Switch/3
  SampleDropOffCmdLogic/1(Out1) -> [SampleDropOffFlag]
  SamplePickUpCmdLogic/1(Out1) -> [SamplePickFlag]
  Delay/1 -> Switch/2
  ActJointAngles/1 -> Planner Subsystem/1(ActJointAngles)
  SampleLoc wrt arm base/1(SamplePos) -> Planner Subsystem/2(SamplePosition)
  Planner Subsystem/2(SamplePickCmd) -> SamplePickUpCmdLogic/1(u)
  Planner Subsystem/3(SampleDropCmd) -> SampleDropOffCmdLogic/1(u)
  [samplePickedSense] -> Planner Subsystem/3(IsSamplePicked)
  [sampleStoredSense] -> Planner Subsystem/4(IsSampleCollected)
  Planner Subsystem/1(DesJointAngles) -> Switch/1
  Planner Subsystem/4(stop) -> Stop Simulation/1
  [RoverAtGoal] -> Delay1/1
  Delay1/1 -> Planner Subsystem/Enable, Delay/1, SampleLoc wrt arm base/1(Enable)
  SampleLocation/1 -> SampleLoc wrt arm base/2(SampleLoc)
